simulink model "DT_NON_IDEAL_INTEGRATOR"  (R2025b)
settings: Solver=VariableStepAuto  StartTime=0.0  StopTime=10.0  RelTol=1e-3
undefined symbols (not defined in the file): Fs
libraries: cstblocks x1, dspobslib x1
settings Model: Creator=divya  LastModifiedBy=divya

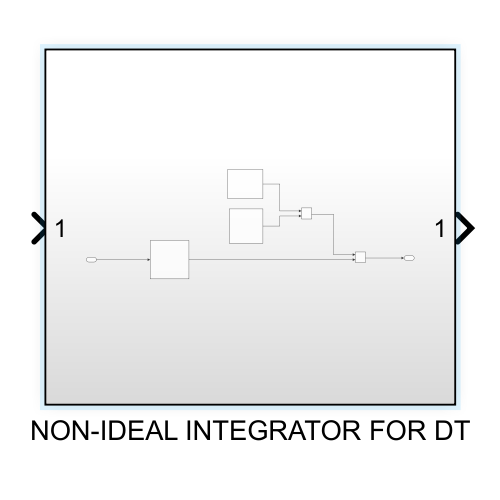
[thumbnail: Simulink's stored preview of the top-level diagram]
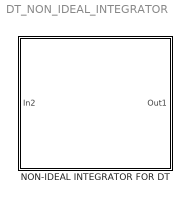
== system DT_NON_IDEAL_INTEGRATOR ==
  NON-IDEAL INTEGRATOR FOR DT : Subsystem

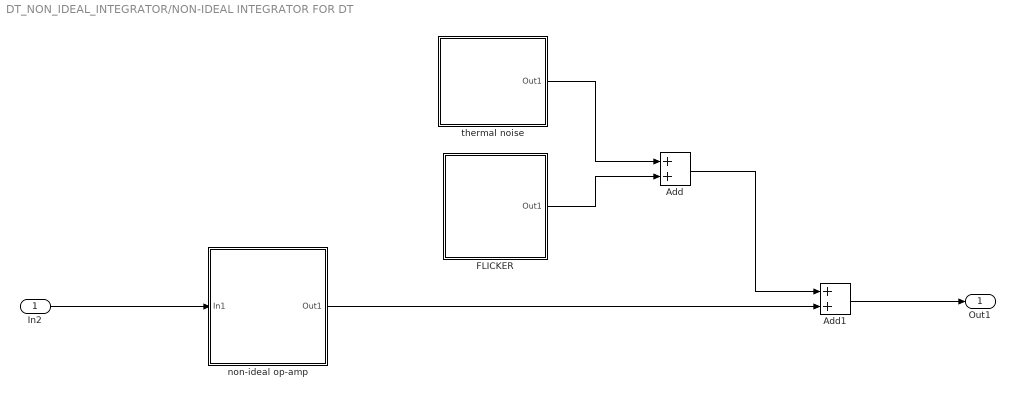
== system DT_NON_IDEAL_INTEGRATOR/NON-IDEAL INTEGRATOR FOR DT ==
  In2 : Inport
  Add : Sum
  Add1 : Sum
  FLICKER : Subsystem
  "non-ideal op-amp " : Subsystem
  thermal noise : Subsystem
  Out1 : Outport
  wires:
  In2/1 -> "non-ideal op-amp "/1(In1)
  Add/1 -> Add1/1
  Add1/1 -> Out1/1
  "non-ideal op-amp "/1(Out1) -> Add1/2
  thermal noise/1(Out1) -> Add/1
  FLICKER/1(Out1) -> Add/2

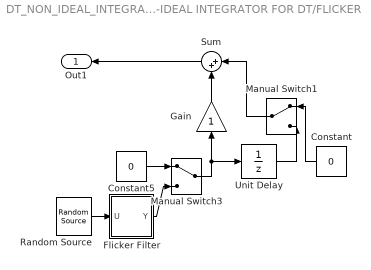
== system DT_NON_IDEAL_INTEGRATOR/NON-IDEAL INTEGRATOR FOR DT/FLICKER ==
  Constant : Constant  Value=0
  Constant5 : Constant  Value=0  SampleTime=1/Fs
  Flicker Filter : Subsystem
  Gain : Gain
  Manual Switch1 : ManualSwitch
  Manual Switch3 : ManualSwitch
  Random Source : dspobslib/Random Source  SrcType=Gaussian  NormMethod=Ziggurat  CltLength=12  MinVal=0  MaxVal=1  MeanVal=0  VarVal=1  RepMode=Not repeatable  rawSeed=1  IsInherit=off  SampMode=Discrete  SampTime=1/Fs  SampFrame=1  DataType=Double  OutComplex=Real  OutputFrames=off
  Sum : Sum  Inputs=|++
  Unit Delay : UnitDelay  SampleTime=1/Fs  HasFrameUpgradeWarning=on
  Out1 : Outport
  wires:
  Manual Switch3/1 -> Gain/1, Unit Delay/1
  Random Source/1 -> Flicker Filter/1(U)
  Unit Delay/1 -> Manual Switch1/2
  Constant5/1 -> Manual Switch3/1
  Constant/1 -> Manual Switch1/1
  Gain/1 -> Sum/2
  Manual Switch1/1 -> Sum/1
  Flicker Filter/1(Y) -> Manual Switch3/2
  Sum/1 -> Out1/1

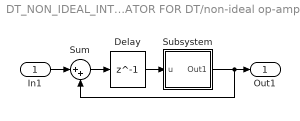
== system DT_NON_IDEAL_INTEGRATOR/NON-IDEAL INTEGRATOR FOR DT/non-ideal op-amp  ==
  In1 : Inport
  Delay : Delay  DelayLength=1  InputProcessing=Columns as channels (frame based)  SampleTime=1/(2e3*128)
  Subsystem : Subsystem
  Sum : Sum  Inputs=|++
  Out1 : Outport
  wires:
  Subsystem/1(Out1) -> Out1/1, Sum/2
  In1/1 -> Sum/1
  Sum/1 -> Delay/1
  Delay/1 -> Subsystem/1(u)

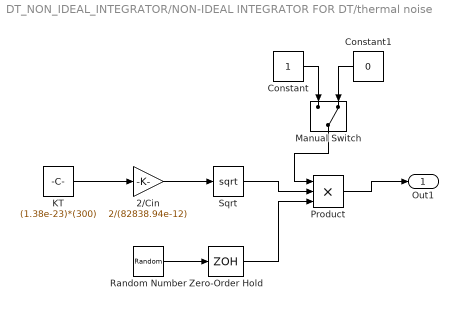
== system DT_NON_IDEAL_INTEGRATOR/NON-IDEAL INTEGRATOR FOR DT/thermal noise ==
  2/Cin : Gain  Gain=2/(82838.94e-12)
  Constant : Constant
  Constant1 : Constant  Value=0
  KT : Constant  Value=(1.38e-23)*(300)
  Manual Switch : ManualSwitch  CurrentSetting=0
  Product : Product  Inputs=3
  Random Number : RandomNumber  SampleTime=0.1
  Sqrt : Sqrt
  Zero-Order Hold : ZeroOrderHold  SampleTime=1/(2e3*128)
  Out1 : Outport
  wires:
  Product/1 -> Out1/1
  Random Number/1 -> Zero-Order Hold/1
  KT/1 -> 2/Cin/1
  2/Cin/1 -> Sqrt/1
  Constant1/1 -> Manual Switch/2
  Constant/1 -> Manual Switch/1
  Zero-Order Hold/1 -> Product/3
  Sqrt/1 -> Product/2
  Manual Switch/1 -> Product/1

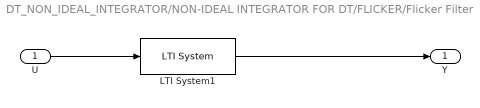
== system DT_NON_IDEAL_INTEGRATOR/NON-IDEAL INTEGRATOR FOR DT/FLICKER/Flicker Filter ==
  U : Inport
  LTI System1 : cstblocks/LTI System  sys=ff_dt  IC=[]  PadeOrder=0
  Y : Outport
  wires:
  LTI System1/1 -> Y/1
  U/1 -> LTI System1/1

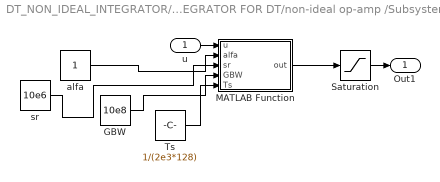
== system DT_NON_IDEAL_INTEGRATOR/NON-IDEAL INTEGRATOR FOR DT/non-ideal op-amp /Subsystem ==
  u : Inport
  GBW : Constant  Value=10e8
  MATLAB Function : MATLAB Function  TreatAsAtomicUnit=on
  Saturation : Saturate  UpperLimit=0.7  LowerLimit=-0.7
  Ts : Constant  Value=1/(2e3*128)
  alfa : Constant
  sr : Constant  Value=10e6
  Out1 : Outport
  wires:
  Ts/1 -> MATLAB Function/5(Ts)
  MATLAB Function/1(out) -> Saturation/1
  alfa/1 -> MATLAB Function/2(alfa)
  GBW/1 -> MATLAB Function/4(GBW)
  sr/1 -> MATLAB Function/3(sr)
  Saturation/1 -> Out1/1
  u/1 -> MATLAB Function/1(u)

== matlab function DT_NON_IDEAL_INTEGRATOR/NON-IDEAL INTEGRATOR FOR DT/non-ideal op-amp /Subsystem/MATLAB Function ==
  data: u input; out output; alfa input; sr input; GBW input; Ts input
function out = slew(u, alfa, sr, GBW, Ts)
% Models the op-amp slew rate for a discrete-time integrator
% u    : input signal amplitude (Vp - Vn)
% alfa : finite gain effect (A0/(1+A0)), ideal op-amp alfa = 1
% sr   : slew rate in V/s
% GBW  : gain-bandwidth of op-amp (Hz)
% Ts   : sample time (s)

tau = 1/(2*pi*GBW);   % time constant
Tmax = Ts/2;           % discrete half-step
slope = alfa * abs(u) / tau;

if slope > sr
    % Op-amp is slewing
    tsl = abs(u)*alfa/sr - tau;   % slewing time
    
    if tsl >= Tmax
        % fully slewing entire half period
        error = abs(u) - sr*Tmax;
    else
        % partial slewing, partial linear region
        texp = Tmax - tsl;
        error = abs(u)*(1-alfa) + (alfa*abs(u) - sr*tsl) * exp(-texp/tau);
    end
    
else
    % Linear region (no slewing)
    texp = Tmax;
    error = abs(u)*(1-alfa) + alfa*abs(u)*exp(-texp/tau);
end

out = u - sign(u)*error;
